simulink model "SBIC2_simulink"  (R2019b)
settings: Solver=VariableStepAuto  StartTime=0.0  StopTime=10  RelTol=1e-3
model workspace (MAT data in the model file):
  PnFrequencyOffset_48 = [30000 100000 1000000 3000000 10000000]
undefined symbols (not defined in the file or in its folder): sigbuilder_block
libraries: fuzblock x1, cstblocks x1
settings Model: Creator=up201809213  LastModifiedBy=up201809213

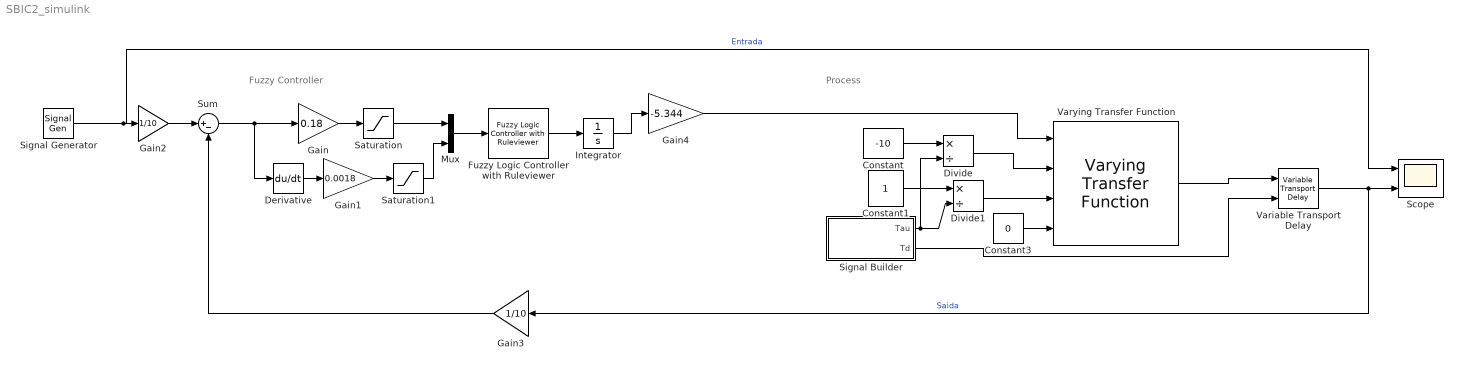
== system SBIC2_simulink ==
  note: Process
  note: Fuzzy Controller
  Constant : Constant  Value=-10
  Constant1 : Constant
  Constant3 : Constant  Value=0
  Derivative : Derivative
  Divide : Product  Inputs=*/
  Divide1 : Product  Inputs=*/
  Fuzzy Logic Controller with Ruleviewer : fuzblock/Fuzzy Logic  Controller  with Ruleviewer  fismatrix=Fuzzy  Ts=2
  Gain : Gain  Gain=0.18
  Gain1 : Gain  Gain=0.0018
  Gain2 : Gain  Gain=1/10
  Gain3 : Gain  Gain=1/10
  Gain4 : Gain  Gain=-5.344
  Integrator : Integrator
  Mux : Mux  Inputs=2
  Saturation : Saturate  UpperLimit=1  LowerLimit=-1
  Saturation1 : Saturate  UpperLimit=1  LowerLimit=-1
  Scope : Scope  NumInputPorts=2
  Signal Generator : SignalGenerator  WaveForm=square  Amplitude=10  Units=rad/sec
  Signal Builder : Subsystem  Tag=STV Subsys  LoadFcn=sigbuilder_block('load');  StartFcn=sigbuilder_block('start');  StopFcn=sigbuilder_block('stop');  ClipboardFcn=sigbuilder_block('clipboard');  mask(Sigbuilder block){tuvar=[0:10]}
      mask help: Simulink:masks:SigbuilderBlock_MD
      mask init:
      | if ~strcmp(get_param(bdroot(gcbh),'SimulationStatus'),'stopped') tuvar = sigbuilder_block('maskInit'); end
      settings: CopyFcn=sigbuilder_block('copy');  DeleteFcn=sigbuilder_block('delete');  ModelCloseFcn=sigbuilder_block('modelClose');  PreSaveFcn=sigbuilder_block('preSave');  PauseFcn=sigbuilder_block('pause');  ContinueFcn=sigbuilder_block('continue');  NameChangeFcn=sigbuilder_block('namechange');  OpenFcn=sigbuilder_block('open',[373.5 43.5 550.5 359.25 ]);  CloseFcn=sigbuilder_block('close');
      mask Display: plot(0, 0, 100, 100,[2, 2, 32, 32, 2], [68, 8, 8, 68, 68],[32, 2], [38, 38], [32, 19, 2],[53, 60, 44], [32, 17, 17, 2],[16, 16, 31, 31]);txt = getActiveGroup(gcbh);text(2, 100, txt,'verticalAlignment', 'top');
  Sum : Sum  Inputs=|+-
  Variable Transport Delay : VariableTransportDelay  VariableDelayType=Variable transport delay  MaximumDelay=10
  Varying Transfer Function : cstblocks/Linear Parameter Varying/Varying Transfer Function  N=1
      settings: SourceProductName=Control System Toolbox
  wires:
  Derivative/1 -> Gain1/1
  Sum/1 -> Derivative/1, Gain/1
  Gain2/1 -> Sum/1
  Mux/1 -> Fuzzy Logic Controller with Ruleviewer/1
  Fuzzy Logic Controller with Ruleviewer/1 -> Integrator/1
  Variable Transport Delay/1 -> Gain3/1, Scope/2  "Saida"
  Gain3/1 -> Sum/2
  Varying Transfer Function/1 -> Variable Transport Delay/1
  Constant3/1 -> Varying Transfer Function/4
  Integrator/1 -> Gain4/1
  Gain4/1 -> Varying Transfer Function/1
  Constant/1 -> Divide/1
  Divide/1 -> Varying Transfer Function/2
  Divide1/1 -> Varying Transfer Function/3
  Constant1/1 -> Divide1/1
  Signal Builder/2(Td) -> Variable Transport Delay/2
  Signal Generator/1 -> Scope/1, Gain2/1  "Entrada"
  Signal Builder/1(Tau) -> Divide1/2, Divide/2
  Gain/1 -> Saturation/1
  Saturation/1 -> Mux/1
  Gain1/1 -> Saturation1/1
  Saturation1/1 -> Mux/2

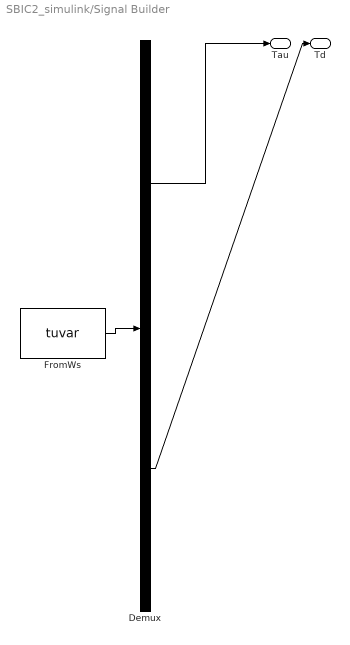
== system SBIC2_simulink/Signal Builder ==
  Demux : Demux  Tag=STV Demux  Outputs=2
  FromWs : FromWorkspace  Tag=STV FromWs  VariableName=tuvar  SampleTime=0
      SigBuilderData=|
      | common.afterFinalStr = 'Extrapolate'
      | common.sampleTime = 0
      | dataSet.timeRange = [0 10]
      | dataSet.name = 'Group 1'
      | sbobj.Groups.Name = 'Group 1'
      | sbobj.Groups.Signals(1).Name = 'Tau'
      | sbobj.Groups.Signals(1).XData = [0 0.5 0.5 1 1 1.5 1.5 2 2 2.5 2.5 3 3 3.5 3.5 4 4 4.5 4.5 5 5 5.5 5.5 6 6 6.5 6.5 7 7 7.5 7.5 8 8 8.5 8.5 9 9 9.5 9.5 10]
      | sbobj.Groups.Signals(1).YData = [0.05 0.05 0.01 0.01 0.05 0.05 0.01 0.01 0.05 0.05 0.01 0.01 0.05 0.05 0.01 0.01 0.05 0.05 0.01 0.01 0.05 0.05 0.01 0.01 0.05 0.05 0.01 0.01 0.05 0.05 0.01 0.01 0.05 0.05 0.01 0.01 0.05 0.05 0.01 0.01]
      | sbobj.Groups.Signals(2).Name = 'Td'
      | sbobj.Groups.Signals(2).XData = [0 0.5 0.5 1 1 1.5 1.5 2 2 2.5 2.5 3 3 3.5 3.5 4 4 4.5 4.5 5 5 5.5 5.5 6 6 6.5 6.5 7 7 7.5 7.5 8 8 8.5 8.5 9 9 9.5 9.5 10]
      | sbobj.Groups.Signals(2).YData = [0.01 0.01 0.003 0.003 0.01 0.01 0.003 0.003 0.01 0.01 0.003 0.003 0.01 0.01 0.003 0.003 0.01 0.01 0.003 0.003 0.01 0.01 0.003 0.003 0.01 0.01 0.003 0.003 0.01 0.01 0.003 0.003 0.01 0.01 0.003 0.003 0.01 0.01 0.003 0.003]
  Tau : Outport  Tag=STV Outport
  Td : Outport  Tag=STV Outport  Port=2
  wires:
  Demux/1 -> Tau/1
  FromWs/1 -> Demux/1
  Demux/2 -> Td/1
